simulink model "puma560_three_model"  (R2015b)
settings: Solver=VariableStepAuto  StartTime=0.0  StopTime=10.0  RelTol=1e-3
values from neighbouring files (symbols this model uses):
  g = -9.8065    [traj_gen.m]
  Ic11 = [Ic11xx -Ic11xy -Ic11xz; -Ic11xy Ic11yy -Ic11yz; -Ic11xz -Ic11yz Ic11zz]    [lagrange_script.m]    (also in lagrange_tao_cal.m; traj_gen.m = [Ic11xx -Ic11xy -Ic11xz)
  Ic22 = [Ic22xx -Ic22xy -Ic22xz; -Ic22xy Ic22yy -Ic22yz; -Ic22xz -Ic22yz Ic22zz]    [lagrange_script.m]    (also in lagrange_tao_cal.m; traj_gen.m = [Ic22xx -Ic22xy -Ic22xz)
  Ic33 = [Ic33xx -Ic33xy -Ic33xz; -Ic33xy Ic33yy -Ic33yz; -Ic33xz -Ic33yz Ic33zz]    [lagrange_script.m]    (also in lagrange_tao_cal.m; traj_gen.m = [Ic33xx -Ic33xy -Ic33xz)
  m1 = 4.43412756    [traj_gen.m]
  m2 = 16.84660904    [traj_gen.m]
  m3 = 4.60251258    [traj_gen.m]
  P112 = [0 d2 0]'    [lagrange_script.m]    (also in lagrange_tao_cal.m; traj_gen.m = [0;d2;0])
  P223 = [a3 0 0]'    [lagrange_script.m]    (also in lagrange_tao_cal.m; traj_gen.m = [a3;0;0])
  P334 = [0 0 0]'    [lagrange_script.m]    (also in lagrange_tao_cal.m; traj_gen.m = [0;0;0])
  Pc11 = [Pc11x;Pc11y;Pc11z]    [lagrange_script.m]    (also in lagrange_tao_cal.m; traj_gen.m)
  Pc22 = [Pc22x;Pc22y;Pc22z]    [lagrange_script.m]    (also in lagrange_tao_cal.m; traj_gen.m)
  Pc33 = [Pc33x;Pc33y;Pc33z]    [lagrange_script.m]    (also in lagrange_tao_cal.m; traj_gen.m)
libraries: mblibv1 x17
settings Model: Creator=jiboc  LastModifiedBy=jiboc
settings SimMechanicsCC: VisDuringSimulation=on

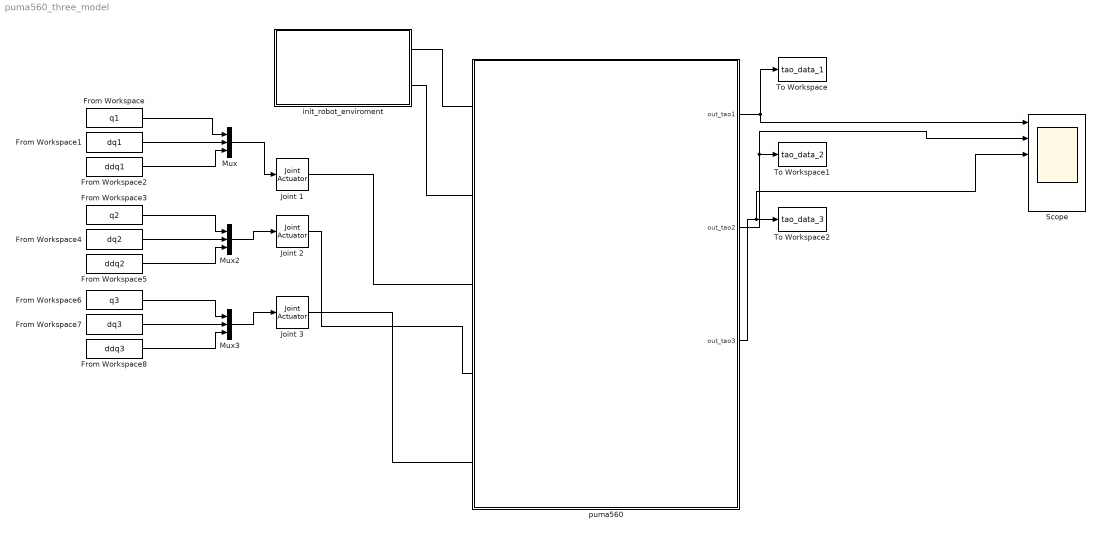
== system puma560_three_model ==
  From Workspace : FromWorkspace  VariableName=q1  SampleTime=0.01
  From Workspace1 : FromWorkspace  VariableName=dq1  SampleTime=0.01
  From Workspace2 : FromWorkspace  VariableName=ddq1  SampleTime=0.01
  From Workspace3 : FromWorkspace  VariableName=q2  SampleTime=0.01
  From Workspace4 : FromWorkspace  VariableName=dq2  SampleTime=0.01
  From Workspace5 : FromWorkspace  VariableName=ddq2  SampleTime=0.01
  From Workspace6 : FromWorkspace  VariableName=q3  SampleTime=0.01
  From Workspace7 : FromWorkspace  VariableName=dq3  SampleTime=0.01
  From Workspace8 : FromWorkspace  VariableName=ddq3  SampleTime=0.01
  Joint 1 : mblibv1/Sensors &  Actuators/Joint Actuator  UpdateFromCAD=off  PhysicalDomain=Mechanical  PortType=blob  ActuationStyle=Motion  AngleUnits=rad  ArcVelocityUnits=rad/s  ArcAccelerationUnits=rad/s^2  CoordPositionUnits=m  VelocityUnits=m/s  AccelerationUnits=m/s^2  ForceUnits=N  TorqueUnits=N*m  ActiveIO=on  Width=3  DialogClass=MechanicalActuatorBlock  Primitive=R1  ReferenceFrame=Absolute (World)
  Joint 2 : mblibv1/Sensors &  Actuators/Joint Actuator  UpdateFromCAD=off  PhysicalDomain=Mechanical  PortType=blob  ActuationStyle=Motion  AngleUnits=rad  ArcVelocityUnits=rad/s  ArcAccelerationUnits=rad/s^2  CoordPositionUnits=m  VelocityUnits=m/s  AccelerationUnits=m/s^2  ForceUnits=N  TorqueUnits=N*m  ActiveIO=on  Width=3  DialogClass=MechanicalActuatorBlock  Primitive=R1  ReferenceFrame=Absolute (World)
  Joint 3 : mblibv1/Sensors &  Actuators/Joint Actuator  UpdateFromCAD=off  PhysicalDomain=Mechanical  PortType=blob  ActuationStyle=Motion  AngleUnits=rad  ArcVelocityUnits=rad/s  ArcAccelerationUnits=rad/s^2  CoordPositionUnits=m  VelocityUnits=m/s  AccelerationUnits=m/s^2  ForceUnits=N  TorqueUnits=N*m  ActiveIO=on  Width=3  DialogClass=MechanicalActuatorBlock  Primitive=R1  ReferenceFrame=Absolute (World)
  Mux : Mux  Inputs=3
  Mux2 : Mux  Inputs=3
  Mux3 : Mux  Inputs=3
  Scope : Scope  NumInputPorts=6
  To Workspace : ToWorkspace  VariableName=tao_data_1  SaveFormat=Timeseries  SampleTime=-1
  To Workspace1 : ToWorkspace  VariableName=tao_data_2  SaveFormat=Timeseries  SampleTime=-1
  To Workspace2 : ToWorkspace  VariableName=tao_data_3  SaveFormat=Timeseries  SampleTime=-1
  "init_robot_enviroment " : Subsystem
  puma560 : Subsystem
  wires:
  From Workspace/1 -> Mux/1
  From Workspace1/1 -> Mux/2
  From Workspace2/1 -> Mux/3
  Mux/1 -> Joint 1/1
  From Workspace3/1 -> Mux2/1
  From Workspace4/1 -> Mux2/2
  From Workspace5/1 -> Mux2/3
  Mux2/1 -> Joint 2/1
  From Workspace6/1 -> Mux3/1
  From Workspace7/1 -> Mux3/2
  From Workspace8/1 -> Mux3/3
  Mux3/1 -> Joint 3/1
  puma560/1(out_tao1) -> To Workspace/1, Scope/1
  puma560/2(out_tao2) -> To Workspace1/1, Scope/2
  puma560/3(out_tao3) -> To Workspace2/1, Scope/3
  connections:
  Joint 1/RConn1 -- puma560/LConn3
  Joint 2/RConn1 -- puma560/LConn4
  puma560/LConn2 -- "init_robot_enviroment "/RConn2
  puma560/LConn1 -- "init_robot_enviroment "/RConn1
  Joint 3/RConn1 -- puma560/LConn5

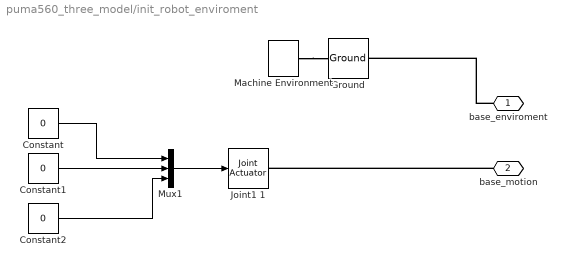
== system puma560_three_model/init_robot_enviroment  ==
  Constant : Constant  Value=0
  Constant1 : Constant  Value=0
  Constant2 : Constant  Value=0
  Ground : mblibv1/Bodies/Ground  UpdateFromCAD=off  LeftPortType=env  RightPortType=workingframe  PhysicalDomain=Mechanical  DialogClass=GroundBlock  CoordPosition=[0 0 0]  CoordPositionUnits=m  StateVectorMgrId=-1  MachineId=[0 0]  ShowEnvPort=on  ParameterChecksum=[3719228666, 1980741807, 273188338, 3448643559]  TopologyChecksum=[1586424466, 1500030333, 874742216, 761425073]
  Joint1 1 : mblibv1/Sensors &  Actuators/Joint Actuator  UpdateFromCAD=off  PhysicalDomain=Mechanical  PortType=blob  ActuationStyle=Motion  AngleUnits=rad  ArcVelocityUnits=rad/s  ArcAccelerationUnits=rad/s^2  CoordPositionUnits=m  VelocityUnits=m/s  AccelerationUnits=m/s^2  ForceUnits=N  TorqueUnits=N*m  ActiveIO=on  Width=3  DialogClass=MechanicalActuatorBlock  Primitive=R1  ReferenceFrame=Absolute (World)
  Machine Environment : mblibv1/Bodies/Machine Environment  PortType=env  PhysicalDomain=Mechanical  DialogTemplateClass=MECH.MachineEnvironment  SyncWhenCopied=off  Gravity=[0 0 -g]  GravityUnits=m/s^2  GravityAsSignal=off  Dimensionality=Auto-detect  AnalysisType=Forward dynamics  LinearAssemblyTolerance=1e-3  LinearAssemblyToleranceUnits=m  AngularAssemblyTolerance=1e-3  AngularAssemblyToleranceUnits=rad  ConstraintSolverType=Stabilizing  ConstraintRelTolerance=1e-4  ConstraintAbsTolerance=1e-4  UseRobustSingularityHandling=off  RedundancyAnalysisToleranceType=Automatically select tolerance  RedundancyAnalysisTolerance=1e-14  StatePerturbationType=Fixed  PerturbationSize=1e-5  VisualizeMachine=on  BodyVisualizationType=Use model default body geometries  BodyColorSelMode=Use model default  DefaultBodyColor=[1 0 0]
  Mux1 : Mux  Inputs=3
  base_enviroment : PMIOPort  Port=1  Side=Right
  base_motion : PMIOPort  Port=2  Side=Right
  wires:
  Constant1/1 -> Mux1/2
  Constant/1 -> Mux1/1
  Constant2/1 -> Mux1/3
  Mux1/1 -> Joint1 1/1
  connections:
  Machine Environment/RConn1 -- Ground/LConn1
  base_motion/RConn1 -- Joint1 1/RConn1
  base_enviroment/RConn1 -- Ground/RConn1

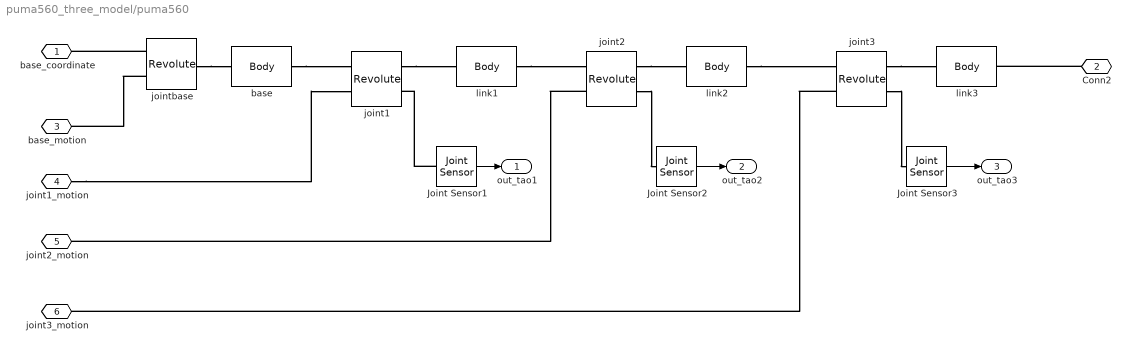
== system puma560_three_model/puma560 ==
  Joint Sensor1 : mblibv1/Sensors &  Actuators/Joint Sensor  UpdateFromCAD=off  PhysicalDomain=Mechanical  PortType=blob  Muxed=on  Pose=off  Angle=off  AngleUnits=deg  ArcVelocity=off  ArcVelocityUnits=deg/s  ArcAcceleration=off  ArcAccelerationUnits=deg/s^2  CoordPosition=on  CoordPositionUnits=m  Velocity=off  VelocityUnits=m/s  Acceleration=off  AccelerationUnits=m/s^2  Quaternion=on  QuaternionDT=off  QuaternionDDT=off  QuaternionUnits=off  OutputVector=[1]  ActiveIO=on  Width=1  DialogClass=MechanicalSensorBlock  Primitive=R1  Force=off  ForceUnits=N  Torque=on  TorqueUnits=N*m  ReferenceFrame=Absolute (World)  ReactionSensedSide=Base  ReactionReferenceFrame=Absolute (World)  ReactionForce=off  ReactionForceUnits=N  ReactionMoment=off  ReactionMomentUnits=N*m
  Joint Sensor2 : mblibv1/Sensors &  Actuators/Joint Sensor  UpdateFromCAD=off  PhysicalDomain=Mechanical  PortType=blob  Muxed=off  Pose=off  Angle=off  AngleUnits=deg  ArcVelocity=off  ArcVelocityUnits=deg/s  ArcAcceleration=off  ArcAccelerationUnits=deg/s^2  CoordPosition=on  CoordPositionUnits=m  Velocity=off  VelocityUnits=m/s  Acceleration=off  AccelerationUnits=m/s^2  Quaternion=on  QuaternionDT=off  QuaternionDDT=off  QuaternionUnits=off  OutputVector=[1]  ActiveIO=on  Width=1  DialogClass=MechanicalSensorBlock  Primitive=R1  Force=off  ForceUnits=N  Torque=on  TorqueUnits=N*m  ReferenceFrame=Absolute (World)  ReactionSensedSide=Base  ReactionReferenceFrame=Absolute (World)  ReactionForce=off  ReactionForceUnits=N  ReactionMoment=off  ReactionMomentUnits=N*m
  Joint Sensor3 : mblibv1/Sensors &  Actuators/Joint Sensor  UpdateFromCAD=off  PhysicalDomain=Mechanical  PortType=blob  Muxed=off  Pose=off  Angle=off  AngleUnits=deg  ArcVelocity=off  ArcVelocityUnits=deg/s  ArcAcceleration=off  ArcAccelerationUnits=deg/s^2  CoordPosition=on  CoordPositionUnits=m  Velocity=off  VelocityUnits=m/s  Acceleration=off  AccelerationUnits=m/s^2  Quaternion=on  QuaternionDT=off  QuaternionDDT=off  QuaternionUnits=off  OutputVector=[1]  ActiveIO=on  Width=1  DialogClass=MechanicalSensorBlock  Primitive=R1  Force=off  ForceUnits=N  Torque=on  TorqueUnits=N*m  ReferenceFrame=Absolute (World)  ReactionSensedSide=Base  ReactionReferenceFrame=Absolute (World)  ReactionForce=off  ReactionForceUnits=N  ReactionMoment=off  ReactionMomentUnits=N*m
  "base " : mblibv1/Bodies/Body  LConnTagsString=CS1  RConnTagsString=CS2  UpdateFromCAD=off  DialogClass=MechanicalBodyBlock  Mass=1  MassUnits=kg  InertiaUnits=kg*m^2  Inertia=eye(3)  Shape=Cylinder  ShapeDims=[1 1]  ShapeUnits=m  ShapeUse=false  Density=1  DensityUnits=kg/m^3  DensityUse=false  GraphicsMode=GFXFILE  GraphicsFileName=E:\003_Robotics\机器人导论\dynamic\Puma650\puma560stl\RobotPart0.STL  BodyColorSelMode=COLORPALETTE  BodyColor=[0.31372 0.31372 0.31372]  AttachedToCS=CS3  CG=Left$CG$[0 0 300]$WORLD$WORLD$mm$[0 0 0]$Euler X-Y-Z$deg$WORLD$false$none  WorkingFrames="Left$CS1$[0 0 0]$World$World$mm$[0 0 0]$Euler X-Y-Z$deg$WORLD$true$none#Right$CS2$[0 0  633.57]$World$World$mm$[0 0 0]$Euler X-Y-Z$deg$WORLD$true$none#Right$CS3$[0 -568 0]$World$World$mm$[0 0 0]$Euler X-Y-Z$deg$WORLD$false$none"  CGPos=[0 0 300]  CGRot=[0 0 0]  CS0Pos=[]  CS0Rot=[]  CS1Pos=[0 0 0]  CS1Rot=[0 0 0]  CS2Pos="[0 0  633.57]"  CS2Rot=[0 0 0]  CS3Pos=[0 -568 0]  CS3Rot=[0 0 0]  CS4Pos=[]  CS4Rot=[]  CS5Pos=[]  CS5Rot=[]  CS6Pos=[]  CS6Rot=[]  CS7Pos=[]  CS7Rot=[]  CS8Pos=[]  CS8Rot=[]  CS9Pos=[]  CS9Rot=[]  CS10Pos=[]  CS10Rot=[]  CS11Pos=[]  CS11Rot=[]  CS12Pos=[]  CS12Rot=[]  CS13Pos=[]  CS13Rot=[]  CS14Pos=[]  CS14Rot=[]  CS15Pos=[]  CS15Rot=[]  CS16Pos=[]  CS16Rot=[]  CS17Pos=[]  CS17Rot=[]  CS18Pos=[]  CS18Rot=[]  CS19Pos=[]  CS19Rot=[]  CS20Pos=[]  CS20Rot=[]
  joint1 : mblibv1/Joints/Revolute  LConnTagsString=__newl0|SA1  RConnTagsString=__newr0|SA1  UpdateFromCAD=off  NumSAPorts=2  CutJoint=off  MarkAsCut=off  Primitives=prismatic  PrimitiveProps=R1$Base$[0 0 1]$revolute  DialogClass=JointBlock  R1Axis=[0 0 1]
  joint2 : mblibv1/Joints/Revolute  LConnTagsString=__newl0|SA1  RConnTagsString=__newr0|SA1  UpdateFromCAD=off  NumSAPorts=2  CutJoint=off  MarkAsCut=off  Primitives=prismatic  PrimitiveProps=R1$Base$[0 0 1]$revolute  DialogClass=JointBlock  R1Axis=[0 0 1]
  joint3 : mblibv1/Joints/Revolute  LConnTagsString=__newl0|SA1  RConnTagsString=__newr0|SA1  UpdateFromCAD=off  NumSAPorts=2  CutJoint=off  MarkAsCut=off  Primitives=prismatic  PrimitiveProps=R1$Base$[0 0 1]$revolute  DialogClass=JointBlock  R1Axis=[0 0 1]
  jointbase : mblibv1/Joints/Revolute  LConnTagsString=__newl0|SA1  RConnTagsString=__newr0  UpdateFromCAD=off  NumSAPorts=1  CutJoint=off  MarkAsCut=off  Primitives=prismatic  PrimitiveProps=R1$World$[0 0 1]$revolute  DialogClass=JointBlock  R1Axis=[0 0 1]
  "link1 " : mblibv1/Bodies/Body  LConnTagsString=CS1  RConnTagsString=CS2  UpdateFromCAD=off  DialogClass=MechanicalBodyBlock  Mass=m1  MassUnits=kg  InertiaUnits=kg*m^2  Inertia=Ic11  Shape=Cylinder  ShapeDims=[1 1]  ShapeUnits=m  ShapeUse=false  Density=1  DensityUnits=kg/m^3  DensityUse=false  GraphicsMode=GFXFILE  GraphicsFileName=E:\003_Robotics\机器人导论\dynamic\Puma650\puma560stl\RobotPart1.STL  BodyColorSelMode=COLORPALETTE  BodyColor=[1 1 0]  AttachedToCS=CS3  CG=Left$CG$Pc11'*1000$CS1$CS1$mm$[0 0 0]$Euler X-Y-Z$deg$CS1$false$none  WorkingFrames=Left$CS1$[0 0 0]$Adjoining$Adjoining$mm$[0 0 0]$Euler X-Y-Z$deg$WORLD$true$none#Right$CS2$P112'*1000$CS1$CS1$mm$[-90 0 0]$Euler X-Y-Z$deg$CS1$true$none#Left$CS3$[0 -568 0]$World$World$mm$[0 0 0]$Euler X-Y-Z$deg$WORLD$false$none  CGPos=Pc11'*1000  CGRot=[0 0 0]  CS0Pos=[]  CS0Rot=[]  CS1Pos=[0 0 0]  CS1Rot=[0 0 0]  CS2Pos=P112'*1000  CS2Rot=[-90 0 0]  CS3Pos=[0 -568 0]  CS3Rot=[0 0 0]  CS4Pos=[]  CS4Rot=[]  CS5Pos=[]  CS5Rot=[]  CS6Pos=[]  CS6Rot=[]  CS7Pos=[]  CS7Rot=[]  CS8Pos=[]  CS8Rot=[]  CS9Pos=[]  CS9Rot=[]  CS10Pos=[]  CS10Rot=[]  CS11Pos=[]  CS11Rot=[]  CS12Pos=[]  CS12Rot=[]  CS13Pos=[]  CS13Rot=[]  CS14Pos=[]  CS14Rot=[]  CS15Pos=[]  CS15Rot=[]  CS16Pos=[]  CS16Rot=[]  CS17Pos=[]  CS17Rot=[]  CS18Pos=[]  CS18Rot=[]  CS19Pos=[]  CS19Rot=[]  CS20Pos=[]  CS20Rot=[]
  link2 : mblibv1/Bodies/Body  LConnTagsString=CS1  RConnTagsString=CS2  UpdateFromCAD=off  DialogClass=MechanicalBodyBlock  Mass=m2  MassUnits=kg  InertiaUnits=kg*m^2  Inertia=Ic22  Shape=Cylinder  ShapeDims=[1 1]  ShapeUnits=m  ShapeUse=false  Density=1  DensityUnits=kg/m^3  DensityUse=false  GraphicsMode=GFXFILE  GraphicsFileName=E:\003_Robotics\机器人导论\dynamic\Puma650\puma560stl\RobotPart2.STL  BodyColorSelMode=COLORPALETTE  BodyColor=[0.87059 0.4902 0]  AttachedToCS=CS3  CG=Left$CG$Pc22'*1000$CS1$CS1$mm$[0 0 0]$Euler X-Y-Z$deg$CS1$false$none  WorkingFrames=Left$CS1$[0 0 0]$Adjoining$Adjoining$mm$[0 0 0]$Euler X-Y-Z$deg$Adjoining$true$none#Right$CS2$P223*1000$CS1$CS1$mm$[0 0 -180]$Euler X-Y-Z$deg$CS1$true$none#Left$CS3$[0 -568 0]$World$World$mm$[0 0 0]$Euler X-Y-Z$deg$World$false$none  CGPos=Pc22'*1000  CGRot=[0 0 0]  CS0Pos=[]  CS0Rot=[]  CS1Pos=[0 0 0]  CS1Rot=[0 0 0]  CS2Pos=P223*1000  CS2Rot=[0 0 -180]  CS3Pos=[0 -568 0]  CS3Rot=[0 0 0]  CS4Pos=[]  CS4Rot=[]  CS5Pos=[]  CS5Rot=[]  CS6Pos=[]  CS6Rot=[]  CS7Pos=[]  CS7Rot=[]  CS8Pos=[]  CS8Rot=[]  CS9Pos=[]  CS9Rot=[]  CS10Pos=[]  CS10Rot=[]  CS11Pos=[]  CS11Rot=[]  CS12Pos=[]  CS12Rot=[]  CS13Pos=[]  CS13Rot=[]  CS14Pos=[]  CS14Rot=[]  CS15Pos=[]  CS15Rot=[]  CS16Pos=[]  CS16Rot=[]  CS17Pos=[]  CS17Rot=[]  CS18Pos=[]  CS18Rot=[]  CS19Pos=[]  CS19Rot=[]  CS20Pos=[]  CS20Rot=[]
  link3 : mblibv1/Bodies/Body  LConnTagsString=CS1  RConnTagsString=CS2  UpdateFromCAD=off  DialogClass=MechanicalBodyBlock  Mass=m3  MassUnits=kg  InertiaUnits=kg*m^2  Inertia=Ic33  Shape=Cylinder  ShapeDims=[1 1]  ShapeUnits=m  ShapeUse=false  Density=1  DensityUnits=kg/m^3  DensityUse=false  GraphicsMode=GFXFILE  GraphicsFileName=E:\003_Robotics\机器人导论\dynamic\Puma650\puma560stl\RobotPart3.STL  BodyColorSelMode=COLORPALETTE  BodyColor=[0 1 0]  AttachedToCS=CS3  CG=Left$CG$Pc33'*1000$CS1$CS1$mm$[0 0 0]$Euler X-Y-Z$deg$CS1$false$none  WorkingFrames=Left$CS1$[0 0 0]$Adjoining$Adjoining$mm$[0 0 0]$Euler X-Y-Z$deg$Adjoining$true$none#Right$CS2$P334'*1000$CS1$CS1$mm$[-90 0 0]$Euler X-Y-Z$deg$CS1$true$none#Left$CS3$[0 -568 0]$World$World$mm$[0 0 0]$Euler X-Y-Z$deg$Adjoining$false$none  CGPos=Pc33'*1000  CGRot=[0 0 0]  CS0Pos=[]  CS0Rot=[]  CS1Pos=[0 0 0]  CS1Rot=[0 0 0]  CS2Pos=P334'*1000  CS2Rot=[-90 0 0]  CS3Pos=[0 -568 0]  CS3Rot=[0 0 0]  CS4Pos=[]  CS4Rot=[]  CS5Pos=[]  CS5Rot=[]  CS6Pos=[]  CS6Rot=[]  CS7Pos=[]  CS7Rot=[]  CS8Pos=[]  CS8Rot=[]  CS9Pos=[]  CS9Rot=[]  CS10Pos=[]  CS10Rot=[]  CS11Pos=[]  CS11Rot=[]  CS12Pos=[]  CS12Rot=[]  CS13Pos=[]  CS13Rot=[]  CS14Pos=[]  CS14Rot=[]  CS15Pos=[]  CS15Rot=[]  CS16Pos=[]  CS16Rot=[]  CS17Pos=[]  CS17Rot=[]  CS18Pos=[]  CS18Rot=[]  CS19Pos=[]  CS19Rot=[]  CS20Pos=[]  CS20Rot=[]
  base_coordinate : PMIOPort  Port=1  Side=Left
  Conn2 : PMIOPort  Port=2  Side=Right
  base_motion : PMIOPort  Port=3  Side=Left
  "joint1_motion " : PMIOPort  Port=4  Side=Left
  joint2_motion : PMIOPort  Port=5  Side=Left
  joint3_motion : PMIOPort  Port=6  Side=Left
  out_tao1 : Outport
  out_tao2 : Outport  Port=2
  out_tao3 : Outport  Port=3
  wires:
  Joint Sensor3/1 -> out_tao3/1
  Joint Sensor2/1 -> out_tao2/1
  Joint Sensor1/1 -> out_tao1/1
  connections:
  jointbase/RConn1 -- "base "/LConn1
  jointbase/LConn1 -- base_coordinate/RConn1
  jointbase/LConn2 -- base_motion/RConn1
  joint3/LConn2 -- joint3_motion/RConn1
  joint3/RConn2 -- Joint Sensor3/LConn1
  Conn2/RConn1 -- link3/RConn1
  link2/RConn1 -- joint3/LConn1
  joint3/RConn1 -- link3/LConn1
  "link1 "/RConn1 -- joint2/LConn1
  joint2/RConn1 -- link2/LConn1
  joint2/RConn2 -- Joint Sensor2/LConn1
  joint2/LConn2 -- joint2_motion/RConn1
  "base "/RConn1 -- joint1/LConn1
  "joint1_motion "/RConn1 -- joint1/LConn2
  Joint Sensor1/LConn1 -- joint1/RConn2
  joint1/RConn1 -- "link1 "/LConn1
